simulink model "System_Architecture"  (R2024b)
settings: Solver=FixedStepDiscrete  StartTime=0.0  StopTime=10.0  RelTol=1e-3
settings Model: Creator=Amin  LastModifiedBy=Amin
settings OptimizationCC: DefaultParameterBehavior=Inlined  EnhancedBackFolding=on  PassReuseOutputArgsAs=Individual arguments  ZeroExternalMemoryAtStartup=off  ZeroInternalMemoryAtStartup=off  OptimizeBlockOrder=speed  DifferentSizesBufferReuse=on  OptimizationCustomize=off  EfficientTunableParamExpr=on
settings DebuggingCC: ParameterTunabilityLossMsg=error
settings SFSimCC: MATLABDynamicMemAlloc=off
settings RTWCC: Description=Embedded Coder  SystemTargetFile=ert.tlc  TemplateMakefile=ert_default_tmf
settings CodeAppCC: ForceParamTrailComments=on  IgnoreCustomStorageClasses=off  OperatorAnnotations=on  SimulinkDataObjDesc=on  SFDataObjDesc=on  InsertBlockDesc=on
settings ERTTargetCC: TargetLangStandard=C99 (ISO)  GenerateSampleERTMain=on  ERTCustomFileTemplate=example_file_process.tlc

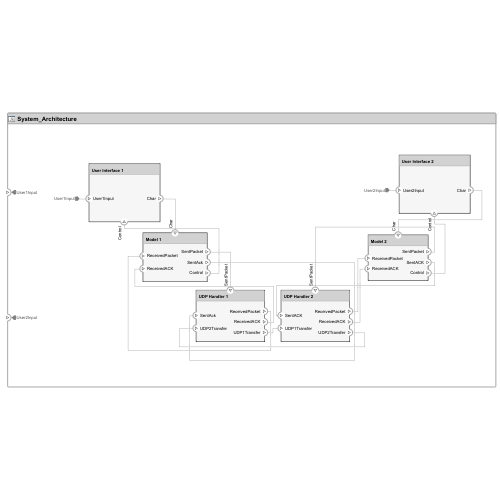
[thumbnail: Simulink's stored preview of the top-level diagram]
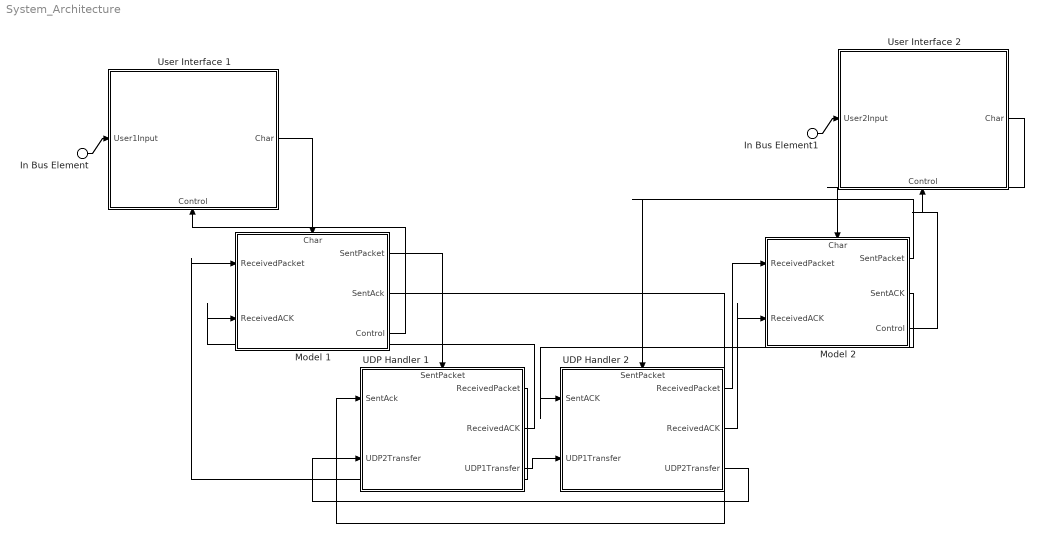
== system System_Architecture ==
  In Bus Element : Inport  PortName=User1Input
  In Bus Element1 : Inport  Port=2  PortName=User2Input
  Model 1 : Subsystem
      settings: PortSchema="{\"entries\":[{\"content\":{\"headerSize\":26,\"margin\":15,\"minimumSpacing\":25,\"sides\":[{\"content\":{\"connectorIds\":[\"In1\",\"In2\"]},\"type\":\"ConnectorPlacement.EquallySpacedRectSide\",\"uuid\":\"4edb8ff1-e7e5-48ac-b271-d2d102bbe1d5\"},{\"content\":{\"connectorIds\":[\"Out1\",\"Out2\",\"Out3\"],\"side\":\"RIGHT\"},\"type\":\"ConnectorPlacement.EquallySpacedRectSide\",\"uuid\":\"60f8fef8-2ea4-4852-8cd6-3c57397af44a\"},{\"content\":{\"connectorIds\":[\"In3\"],\"side\":\"TOP\"},\"type\":\"ConnectorPlacement.EquallySpacedRectSide\",\"uuid\":\"73e34a08-2d41-449e-8ca4-cf0707e80820\"},{\"content\":{\"side\":\"BOTTOM\"},\"type\":\"ConnectorPlacement.EquallySpacedRectSide\",\"uuid\":\"c75753dd-5f90-4377-8318-b222503906dc\"}]},\"type\":\"ConnectorPlacement.EquallySpacedConnector\",\"uuid\":\"582517f9-0612-4b15-9736-2f3b36a5d53f\"}],\"packageUris\":[\"http://schema.mathworks.com/mf0/Connector/R2020b\"],\"version\":\"1.0\"}"
  Model 2 : Subsystem
      settings: PortSchema="{\"entries\":[{\"content\":{\"headerSize\":26,\"margin\":15,\"minimumSpacing\":25,\"sides\":[{\"content\":{\"connectorIds\":[\"In2\",\"In1\"]},\"type\":\"ConnectorPlacement.EquallySpacedRectSide\",\"uuid\":\"4edb8ff1-e7e5-48ac-b271-d2d102bbe1d5\"},{\"content\":{\"connectorIds\":[\"Out1\",\"Out2\",\"Out3\"],\"side\":\"RIGHT\"},\"type\":\"ConnectorPlacement.EquallySpacedRectSide\",\"uuid\":\"60f8fef8-2ea4-4852-8cd6-3c57397af44a\"},{\"content\":{\"connectorIds\":[\"In3\"],\"side\":\"TOP\"},\"type\":\"ConnectorPlacement.EquallySpacedRectSide\",\"uuid\":\"73e34a08-2d41-449e-8ca4-cf0707e80820\"},{\"content\":{\"side\":\"BOTTOM\"},\"type\":\"ConnectorPlacement.EquallySpacedRectSide\",\"uuid\":\"8987c667-9623-4988-acd5-943fb1986598\"}]},\"type\":\"ConnectorPlacement.EquallySpacedConnector\",\"uuid\":\"582517f9-0612-4b15-9736-2f3b36a5d53f\"}],\"packageUris\":[\"http://schema.mathworks.com/mf0/Connector/R2020b\"],\"version\":\"1.0\"}"
  UDP Handler 1 : Subsystem
      settings: PortSchema="{\"entries\":[{\"content\":{\"headerSize\":26,\"margin\":15,\"minimumSpacing\":25,\"sides\":[{\"content\":{\"connectorIds\":[\"In1\",\"In3\"]},\"type\":\"ConnectorPlacement.EquallySpacedRectSide\",\"uuid\":\"4edb8ff1-e7e5-48ac-b271-d2d102bbe1d5\"},{\"content\":{\"connectorIds\":[\"Out1\",\"Out2\",\"Out3\"],\"side\":\"RIGHT\"},\"type\":\"ConnectorPlacement.EquallySpacedRectSide\",\"uuid\":\"60f8fef8-2ea4-4852-8cd6-3c57397af44a\"},{\"content\":{\"connectorIds\":[\"In2\"],\"side\":\"TOP\"},\"type\":\"ConnectorPlacement.EquallySpacedRectSide\",\"uuid\":\"73e34a08-2d41-449e-8ca4-cf0707e80820\"}]},\"type\":\"ConnectorPlacement.EquallySpacedConnector\",\"uuid\":\"582517f9-0612-4b15-9736-2f3b36a5d53f\"}],\"packageUris\":[\"http://schema.mathworks.com/mf0/Connector/R2020b\"],\"version\":\"1.0\"}"
  UDP Handler 2 : Subsystem
      settings: PortSchema="{\"entries\":[{\"content\":{\"headerSize\":26,\"margin\":15,\"minimumSpacing\":25,\"sides\":[{\"content\":{\"connectorIds\":[\"In1\",\"In3\"]},\"type\":\"ConnectorPlacement.EquallySpacedRectSide\",\"uuid\":\"4edb8ff1-e7e5-48ac-b271-d2d102bbe1d5\"},{\"content\":{\"connectorIds\":[\"Out1\",\"Out2\",\"Out3\"],\"side\":\"RIGHT\"},\"type\":\"ConnectorPlacement.EquallySpacedRectSide\",\"uuid\":\"60f8fef8-2ea4-4852-8cd6-3c57397af44a\"},{\"content\":{\"connectorIds\":[\"In2\"],\"side\":\"TOP\"},\"type\":\"ConnectorPlacement.EquallySpacedRectSide\",\"uuid\":\"73e34a08-2d41-449e-8ca4-cf0707e80820\"}]},\"type\":\"ConnectorPlacement.EquallySpacedConnector\",\"uuid\":\"582517f9-0612-4b15-9736-2f3b36a5d53f\"}],\"packageUris\":[\"http://schema.mathworks.com/mf0/Connector/R2020b\"],\"version\":\"1.0\"}"
  User Interface 1 : Subsystem
      settings: PortSchema="{\"entries\":[{\"content\":{\"headerSize\":26,\"margin\":15,\"minimumSpacing\":25,\"sides\":[{\"content\":{\"connectorIds\":[\"In2\"]},\"type\":\"ConnectorPlacement.EquallySpacedRectSide\",\"uuid\":\"4edb8ff1-e7e5-48ac-b271-d2d102bbe1d5\"},{\"content\":{\"connectorIds\":[\"Out1\"],\"side\":\"RIGHT\"},\"type\":\"ConnectorPlacement.EquallySpacedRectSide\",\"uuid\":\"60f8fef8-2ea4-4852-8cd6-3c57397af44a\"},{\"content\":{\"side\":\"TOP\"},\"type\":\"ConnectorPlacement.EquallySpacedRectSide\",\"uuid\":\"73e34a08-2d41-449e-8ca4-cf0707e80820\"},{\"content\":{\"connectorIds\":[\"In1\"],\"side\":\"BOTTOM\"},\"type\":\"ConnectorPlacement.EquallySpacedRectSide\",\"uuid\":\"c1c38803-3ae6-4c81-b7e8-4891d6b4434b\"}]},\"type\":\"ConnectorPlacement.EquallySpacedConnector\",\"uuid\":\"582517f9-0612-4b15-9736-2f3b36a5d53f\"}],\"packageUris\":[\"http://schema.mathworks.com/mf0/Connector/R2020b\"],\"version\":\"1.0\"}"
  User Interface 2 : Subsystem
      settings: PortSchema="{\"entries\":[{\"content\":{\"headerSize\":26,\"margin\":15,\"minimumSpacing\":25,\"sides\":[{\"content\":{\"connectorIds\":[\"In1\"]},\"type\":\"ConnectorPlacement.EquallySpacedRectSide\",\"uuid\":\"4edb8ff1-e7e5-48ac-b271-d2d102bbe1d5\"},{\"content\":{\"connectorIds\":[\"Out1\"],\"side\":\"RIGHT\"},\"type\":\"ConnectorPlacement.EquallySpacedRectSide\",\"uuid\":\"60f8fef8-2ea4-4852-8cd6-3c57397af44a\"},{\"content\":{\"side\":\"TOP\"},\"type\":\"ConnectorPlacement.EquallySpacedRectSide\",\"uuid\":\"73e34a08-2d41-449e-8ca4-cf0707e80820\"},{\"content\":{\"connectorIds\":[\"In2\"],\"side\":\"BOTTOM\"},\"type\":\"ConnectorPlacement.EquallySpacedRectSide\",\"uuid\":\"74686dc6-5040-45be-bc12-3166f32c71ce\"}]},\"type\":\"ConnectorPlacement.EquallySpacedConnector\",\"uuid\":\"582517f9-0612-4b15-9736-2f3b36a5d53f\"}],\"packageUris\":[\"http://schema.mathworks.com/mf0/Connector/R2020b\"],\"version\":\"1.0\"}"
  wires:
  UDP Handler 1/3(UDP1Transfer) -> UDP Handler 2/3(UDP1Transfer)
  UDP Handler 2/3(UDP2Transfer) -> UDP Handler 1/3(UDP2Transfer)
  User Interface 1/1(Char) -> Model 1/3(Char)
  Model 1/1(SentPacket) -> UDP Handler 1/2(SentPacket)
  Model 2/1(SentPacket) -> UDP Handler 2/2(SentPacket)
  User Interface 2/1(Char) -> Model 2/3(Char)
  UDP Handler 2/2(ReceivedACK) -> Model 2/1(ReceivedACK)
  Model 2/3(Control) -> User Interface 2/2(Control)
  In Bus Element/1 -> User Interface 1/2(User1Input)
  In Bus Element1/1 -> User Interface 2/1(User2Input)
  UDP Handler 1/2(ReceivedACK) -> Model 1/2(ReceivedACK)
  Model 1/3(Control) -> User Interface 1/1(Control)
  UDP Handler 2/1(ReceivedPacket) -> Model 2/2(ReceivedPacket)
  Model 2/2(SentACK) -> UDP Handler 2/1(SentACK)
  UDP Handler 1/1(ReceivedPacket) -> Model 1/1(ReceivedPacket)
  Model 1/2(SentAck) -> UDP Handler 1/1(SentAck)

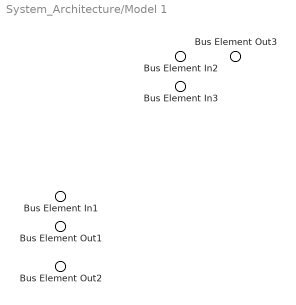
== system System_Architecture/Model 1 ==
  Bus Element In3 : Inport  PortName=ReceivedPacket
  Bus Element In2 : Inport  Port=2  PortName=ReceivedACK
  Bus Element In1 : Inport  Port=3  PortName=Char
  Bus Element Out1 : Outport  PortName=SentPacket
  Bus Element Out3 : Outport  Port=2  PortName=SentAck
  Bus Element Out2 : Outport  Port=3  PortName=Control

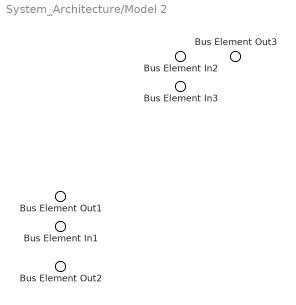
== system System_Architecture/Model 2 ==
  Bus Element In2 : Inport  PortName=ReceivedACK
  Bus Element In3 : Inport  Port=2  PortName=ReceivedPacket
  Bus Element In1 : Inport  Port=3  PortName=Char
  Bus Element Out1 : Outport  PortName=SentPacket
  Bus Element Out3 : Outport  Port=2  PortName=SentACK
  Bus Element Out2 : Outport  Port=3  PortName=Control

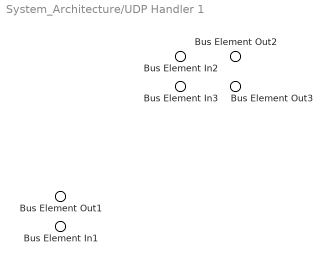
== system System_Architecture/UDP Handler 1 ==
  Bus Element In3 : Inport  PortName=SentAck
  Bus Element In2 : Inport  Port=2  PortName=SentPacket
  Bus Element In1 : Inport  Port=3  PortName=UDP2Transfer
  Bus Element Out3 : Outport  PortName=ReceivedPacket
  Bus Element Out2 : Outport  Port=2  PortName=ReceivedACK
  Bus Element Out1 : Outport  Port=3  PortName=UDP1Transfer

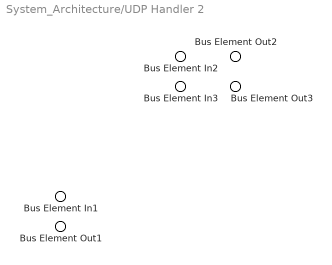
== system System_Architecture/UDP Handler 2 ==
  Bus Element In3 : Inport  PortName=SentACK
  Bus Element In2 : Inport  Port=2  PortName=SentPacket
  Bus Element In1 : Inport  Port=3  PortName=UDP1Transfer
  Bus Element Out3 : Outport  PortName=ReceivedPacket
  Bus Element Out2 : Outport  Port=2  PortName=ReceivedACK
  Bus Element Out1 : Outport  Port=3  PortName=UDP2Transfer

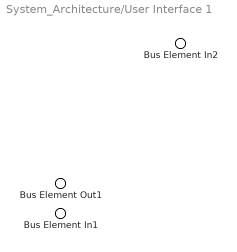
== system System_Architecture/User Interface 1 ==
  Bus Element In2 : Inport  PortName=Control
  Bus Element In1 : Inport  Port=2  PortName=User1Input
  Bus Element Out1 : Outport  PortName=Char

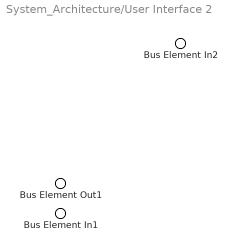
== system System_Architecture/User Interface 2 ==
  Bus Element In2 : Inport  PortName=User2Input
  Bus Element In1 : Inport  Port=2  PortName=Control
  Bus Element Out1 : Outport  PortName=Char
